simulink model "Main1"  (R2017b)
settings: Solver=ode15s  StartTime=0.0  StopTime=t_end  FixedStep=.0001  MaxStep=st  RelTol=1e-3  EnableMultiTasking=on
values from neighbouring files (symbols this model uses):
  A = eye(16,16)    [full_input_list.m]
  B = zeros(16,1)    [full_input_list.m]
  C = blkdiag(eye(3,3),zeros(3,3),eye(10,10))    [full_input_list.m]
  deltaT = 0.00001    (= 1e-05)    [full_input_list.m]
  H = C    [full_input_list.m]
  I_UD = [0.032808359, 0.000617048, 0.000049185;      0.000617048, 0.032531573, 0.000060042;      0.000049185, 0.000060042, 0.007799591]    [full_input_list.m]
  kd = 0.5    [full_input_list.m]    (also in initACS.m = 0.01)
  kd_UD_detumble = 6e-3    (= 0.006)    [full_input_list.m]
  kd_UD_slew = epsilon_UD_slew*.3    (= 0.003)    [full_input_list.m]
  kd_UD_spinUp = epsilon_UD_spinUp*0.025    (= 0.00025)    [full_input_list.m]
  kp = 1    [full_input_list.m]    (also in initACS.m = 0.01)
  kp_UD_slew = epsilon_UD_slew^2*.01    (= 1e-06)    [full_input_list.m]
  kp_UD_spinUp = epsilon_UD_spinUp^2*.05    (= 5e-06)    [full_input_list.m]
  magMomentMax_B = sat2CoilArea.*sat2n.*currentMax_B    [full_input_list.m]
  omega_cmd_N = 1e-1*[1 1 -.6]'    [full_input_list.m]
  omega_spinUp_MAG = 0.05    [full_input_list.m]
  OpModes = [0 0 0]    [full_input_list.m]
  OpTimes = [0 1 2]    [full_input_list.m]
  q4_cmd_init = [q4_cmd_init(2:4); q4_cmd_init(1)]    [full_input_list.m]
  Q_k = zeros(16,16)    [full_input_list.m]
  R = R_k    [full_input_list.m]
  sat2CoilArea = 0.8*[0.02; 0.02; 0.01]    [full_input_list.m]
  sat2n = [0; 100; 100]    [full_input_list.m]
  sat2Resistance = sat2WireLength.*sat2WireResistivity./sat2WireArea    [full_input_list.m]
  SeperationTime = 30000    [full_input_list.m]
  spinAxis_B = [1 0 0]    [full_input_list.m]
  st = 1/freq    (= 0.0125)    [full_input_list.m]    (also in initSimulink.m)
  u_k = zeros(16,1)    [full_input_list.m]
  w_k = zeros(16,1)    [full_input_list.m]
  Z_k = zeros(16,1)    [full_input_list.m]
undefined symbols (not defined in the file or in its folder): DiscIntNeverNeededParam, G_igrf, gyro_DCM_BS, H_igrf, I_B, IAU, Kschmidt, mag_variance, R_mean
libraries: aerolibutil x36, vrlib x31, SimMainLibrary x27, simulink x22, dspmathops x6, sharedtransform x4, sharedutil x2, dspinverses x2, dspmtrx3 x1, aerolibtransform2 x1, aerolibgravity2 x1, lib_violet_env x1
(part 3 of 3)

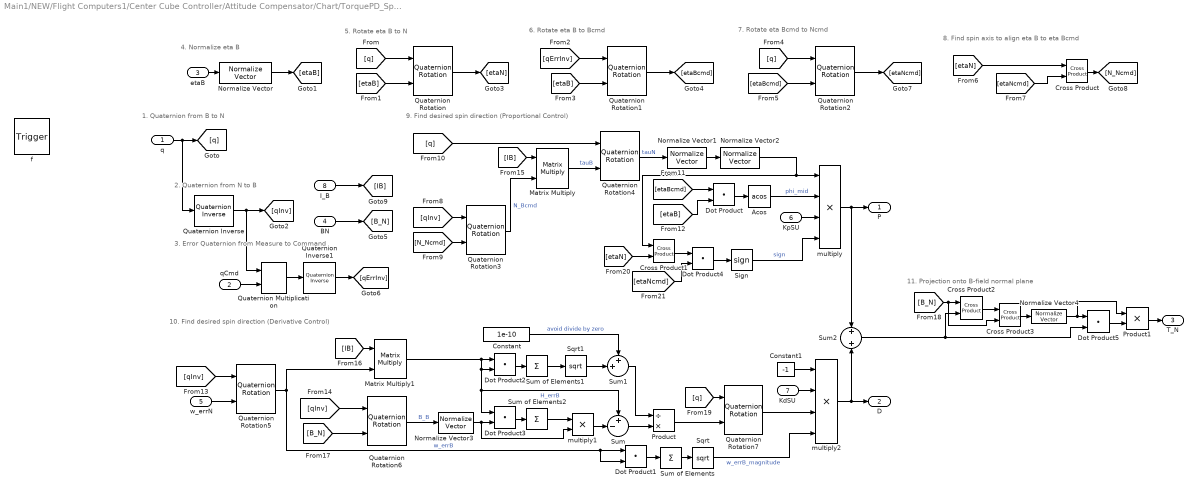
== system Main1/NEW/Flight Computers1/Center Cube Controller/Attitude Compensator/Chart/TorquePD_SpinUp ==
  note: 1. Quaternion from B to N
  note: 5. Rotate eta B to N
  note: 2. Quaternion from N to B
  note: 3. Error Quaternion from Measure to Command
  note: 6. Rotate eta B to Bcmd
  note: 7. Rotate eta Bcmd to Ncmd
  note: 8. Find spin axis to align eta B to eta Bcmd
  note: 9. Find desired spin direction (Proportional Control)
  note: 10. Find desired spin direction (Derivative Control)
  note: 4. Normalize eta B
  note: 11. Projection onto B-field normal plane
  q : Inport
  qCmd : Inport  Port=2
  etaB : Inport  Port=3
  BN : Inport  Port=4
  w_errN : Inport  Port=5
  KpSU : Inport  Port=6
  KdSU : Inport  Port=7
  I_B : Inport  Port=8
  f : TriggerPort  TriggerType=function-call  VariantControl=(inherit)
      settings: CopyFcn=Stateflow.SLINSF.SimulinkMan.removeBlockPreDeleteFcn  PreDeleteFcn=Stateflow.SLINSF.SimulinkMan.unsafePredeleteFcn
  Acos : Trigonometry  Operator=acos
  Constant : Constant  Value=1e-10
  Constant1 : Constant  Value=-1
  Cross Product{,1..3} (4 alike) : vrlib/Utilities/Cross Product
      settings: SourceProductBaseCode=VR
  Dot Product{,1..5} (6 alike) : DotProduct  InputSameDT=on  OutDataTypeStr=Inherit: Inherit via internal rule
  Matrix Multiply : Product  Multiplication=Matrix(*)
  Matrix Multiply1 : Product  Multiplication=Matrix(*)
  Normalize Vector{,1..4} (5 alike) : vrlib/Utilities/Normalize Vector  maxzero=0
      settings: SourceProductName=Simulink 3D Animation  SourceProductBaseCode=VR
  Product : Product  Inputs=/*
  Product1 : Product
  Quaternion Inverse : aerolibutil/Quaternion Inverse
      settings: SourceProductName=Aerospace Blockset
  Quaternion Inverse1 : aerolibutil/Quaternion Inverse
      settings: SourceProductName=Aerospace Blockset
  Quaternion Multiplication : aerolibutil/Quaternion Multiplication
  Quaternion Rotation{,1..7} (8 alike) : aerolibutil/Quaternion Rotation
  Sign : Signum
  Sqrt : Sqrt  SaturateOnIntegerOverflow=on
  Sqrt1 : Sqrt  SaturateOnIntegerOverflow=on
  Sum : Sum  Inputs=+-|
  Sum of Elements : Sum  Inputs=+
  Sum of Elements1 : Sum  Inputs=+
  Sum of Elements2 : Sum  Inputs=+
  Sum1 : Sum  Inputs=++|
  Sum2 : Sum
  multiply : Product  Inputs=****
  multiply1 : Product  Inputs=**
  multiply2 : Product  Inputs=****
  P : Outport
  D : Outport  Port=2
  T_N : Outport  Port=3
  wires:
  etaB/1 -> Normalize Vector/1
  Quaternion Rotation/1 -> [etaN]
  q/1 -> [q], Quaternion Inverse/1
  [q] -> Quaternion Rotation/1
  Normalize Vector/1 -> [etaB]
  [etaB] -> Quaternion Rotation/2
  Quaternion Inverse/1 -> Quaternion Multiplication/1, [qInv]
  [qErrInv] -> Quaternion Rotation1/1
  [etaB] -> Quaternion Rotation1/2
  Quaternion Rotation1/1 -> [etaBcmd]
  qCmd/1 -> Quaternion Multiplication/2
  Quaternion Multiplication/1 -> Quaternion Inverse1/1
  Quaternion Inverse1/1 -> [qErrInv]
  [q] -> Quaternion Rotation2/1
  [etaBcmd] -> Quaternion Rotation2/2
  Quaternion Rotation2/1 -> [etaNcmd]
  [etaN] -> Cross Product/1
  [etaNcmd] -> Cross Product/2
  Cross Product/1 -> [N_Ncmd]
  Quaternion Rotation3/1 -> Matrix Multiply/2  "N_Bcmd"
  [N_Ncmd] -> Quaternion Rotation3/2
  [qInv] -> Quaternion Rotation3/1
  [q] -> Quaternion Rotation4/1
  Matrix Multiply/1 -> Quaternion Rotation4/2  "tauB"
  Quaternion Rotation4/1 -> Normalize Vector1/1  "tauN"
  Normalize Vector1/1 -> Normalize Vector2/1
  Normalize Vector2/1 -> Cross Product1/1, multiply/1
  Dot Product/1 -> Acos/1
  [etaB] -> Dot Product/2
  [etaBcmd] -> Dot Product/1
  Acos/1 -> multiply/2  "phi_mid"
  KpSU/1 -> multiply/3
  multiply/1 -> P/1, Sum2/1
  [qInv] -> Quaternion Rotation5/1
  w_errN/1 -> Quaternion Rotation5/2
  [qInv] -> Quaternion Rotation6/1
  Quaternion Rotation6/1 -> Normalize Vector3/1  "B_B"
  I_B/1 -> [IB]
  [IB] -> Matrix Multiply/1
  [IB] -> Matrix Multiply1/1
  Quaternion Rotation5/1 -> Dot Product1/1, Dot Product1/2, Matrix Multiply1/2  "w_errB"
  Normalize Vector3/1 -> Dot Product3/2, multiply1/2
  Constant/1 -> Sum1/1  "avoid divide by zero"
  [q] -> Quaternion Rotation7/1
  Sum/1 -> Product/2
  Sum1/1 -> Product/1
  Product/1 -> Quaternion Rotation7/2
  Sqrt1/1 -> Sum1/2
  Matrix Multiply1/1 -> Sum/1, Dot Product3/1, Dot Product2/2, Dot Product2/1  "H_errB"
  Dot Product1/1 -> Sum of Elements/1
  Sum of Elements/1 -> Sqrt/1
  Sum of Elements1/1 -> Sqrt1/1
  Dot Product2/1 -> Sum of Elements1/1
  [etaN] -> Cross Product1/2
  Cross Product1/1 -> Dot Product4/1
  [etaNcmd] -> Dot Product4/2
  Dot Product4/1 -> Sign/1
  Sign/1 -> multiply/4  "sign"
  multiply1/1 -> Sum/2
  Dot Product3/1 -> Sum of Elements2/1
  Sum of Elements2/1 -> multiply1/1
  Quaternion Rotation7/1 -> multiply2/3
  KdSU/1 -> multiply2/2
  Constant1/1 -> multiply2/1
  multiply2/1 -> D/1, Sum2/2
  Sqrt/1 -> multiply2/4  "w_errB_magnitude"
  Normalize Vector4/1 -> Product1/1, Dot Product5/1
  Cross Product2/1 -> Cross Product3/1
  [B_N] -> Cross Product2/1, Cross Product3/2
  Cross Product3/1 -> Normalize Vector4/1
  Sum2/1 -> Cross Product2/2, Dot Product5/2
  Product1/1 -> T_N/1
  Dot Product5/1 -> Product1/2
  BN/1 -> [B_N]
  [B_N] -> Quaternion Rotation6/2

== system Main1/NEW/Flight Computers1/Center Cube Controller/Attitude Compensator/Commanded state/Quaternion Integration ==
  w_N : Inport
  Integrator1 : Integrator  InitialCondition=q4_cmd_init
  q_normalize : Subsystem
  qderiv : Subsystem
  q4 : Outport
  wires:
  w_N/1 -> qderiv/1(w)
  q_normalize/1(q_out) -> qderiv/2(q), q4/1
  Integrator1/1 -> q_normalize/1(q_in)
  qderiv/1(qd) -> Integrator1/1

== system Main1/NEW/Flight Computers1/Center Cube Controller/Attitude Compensator/Deployed Modes (switch)1/Default ==
  Action Port : ActionPort  ActionType=default
  Constant : Constant  Value=[ 0 0 0 ]
  Out1 : Outport
  wires:
  Constant/1 -> Out1/1

== system Main1/NEW/Flight Computers1/Center Cube Controller/Attitude Compensator/Deployed Modes (switch)1/Seek EKF Convergence ==
  Action Port : ActionPort  ActionType=case
  Constant : Constant  Value=[ 0 0 0 ]
  Out1 : Outport
  wires:
  Constant/1 -> Out1/1

== system Main1/NEW/Flight Computers1/Center Cube Controller/Attitude Compensator/Deployed Modes (switch)1/Spin-Up Slew ==
  note: Regulator
      | - q_target = [0 0 0 1]
      | - w_target = [0 0 0]
  q : Inport
  w : Inport  Port=2
  Action Port : ActionPort  ActionType=case
  Add : Sum
  Gain : Gain  Gain=-1
  Gain1 : Gain  Gain=kp
  Gain2 : Gain  Gain=-1
  Gain3 : Gain  Gain=kd
  Quaternion Inverse : aerolibutil/Quaternion Inverse
      settings: SourceProductName=Aerospace Blockset
  Quaternion Multiplication : aerolibutil/Quaternion Multiplication
  Selector : Selector  InputPortWidth=4  IndexOptions=Index vector (dialog)  Indices=[1 2 3]  OutputSizes=1
  Target q : Constant  Value=[ 0 0 0 1 ]
  tau : Outport
  wires:
  Gain2/1 -> Add/2
  Gain/1 -> Add/1
  Add/1 -> tau/1
  w/1 -> Gain3/1
  Gain3/1 -> Gain2/1
  Gain1/1 -> Gain/1
  Selector/1 -> Gain1/1
  Quaternion Multiplication/1 -> Selector/1
  Target q/1 -> Quaternion Inverse/1
  Quaternion Inverse/1 -> Quaternion Multiplication/2
  q/1 -> Quaternion Multiplication/1

== system Main1/NEW/Flight Computers1/Center Cube Controller/Attitude Compensator/Not Deployed Modes (switch)/Detumbling Slew ==
  note: Regulator
      | - q_target = [0 0 0 1]
      | - w_target = [0 0 0]
  note: Markley Regulator
      | This regulator takes the current directional quaterion vector, the target quaterion, the intertial matrix, and the current angular velocity to determine the required torque necessary to the slew.
      |
      | The equation is 7.8 listed on page 290 of Fundamentals of Spacecraft Attitude Determination and Control. The input I is currently not defined. Also important to the equation is equation 7.2
  q_BN : Inport
  w_BN : Inport  Port=2
  "Inertia " : Inport  Port=3
  Action Port : ActionPort
  3x3 Cross Product : sharedutil/3x3 Cross Product
      settings: SourceProductBaseCode=AE
  Add : Sum  Inputs=+++
  Gain : Gain  Gain=-1
  Gain1 : Gain  Gain=kp
  Gain2 : Gain  Gain=-1
  Gain3 : Gain  Gain=kd
  Gain4 : Gain  Gain=-1
  Product : Product  Multiplication=Matrix(*)
  Quaternion Inverse : aerolibutil/Quaternion Inverse
      settings: SourceProductName=Aerospace Blockset
  Quaternion Multiplication : aerolibutil/Quaternion Multiplication
  Selector : Selector  InputPortWidth=4  IndexOptions=Index vector (dialog)  Indices=[1 2 3]  OutputSizes=1
  Target q : Constant  Value=[ 0 0 0 1 ]
  tau : Outport
  wires:
  q_BN/1 -> Quaternion Multiplication/1
  Quaternion Inverse/1 -> Quaternion Multiplication/2
  Target q/1 -> Quaternion Inverse/1
  Quaternion Multiplication/1 -> Selector/1
  Selector/1 -> Gain1/1
  Gain1/1 -> Gain/1
  Gain3/1 -> Gain2/1
  w_BN/1 -> 3x3 Cross Product/1, Gain3/1, Product/2
  Add/1 -> tau/1
  Gain/1 -> Add/1
  Gain2/1 -> Add/2
  "Inertia "/1 -> Product/1
  Product/1 -> 3x3 Cross Product/2
  3x3 Cross Product/1 -> Gain4/1
  Gain4/1 -> Add/3

== system Main1/NEW/Flight Computers1/Center Cube Controller/Attitude Compensator/Not Deployed Modes (switch)/Inital Spin Up ==
  note: Regulator
      | - q_target = [0 0 0 1]
      | - w_target = [0 0 0]
  note: Markley Regulator
      | This regulator takes the current directional quaterion vector, the target quaterion, the intertial matrix, and the current angular velocity to determine the required torque necessary to the slew.
      |
      | The equation is 7.8 listed on page 290 of Fundamentals of Spacecraft Attitude Determination and Control. The input I is currently not defined. Also important to the equation is equation 7.2
  q_BN : Inport
  w : Inport  Port=2
  "I " : Inport  Port=3
  Action Port : ActionPort
  3x3 Cross Product : sharedutil/3x3 Cross Product
      settings: SourceProductBaseCode=AE
  Add : Sum  Inputs=+++
  Gain : Gain  Gain=-1
  Gain1 : Gain  Gain=kp
  Gain2 : Gain  Gain=-1
  Gain3 : Gain  Gain=kd
  Gain4 : Gain  Gain=-1
  Product : Product  Multiplication=Matrix(*)
  Quaternion Inverse : aerolibutil/Quaternion Inverse
      settings: SourceProductName=Aerospace Blockset
  Quaternion Multiplication : aerolibutil/Quaternion Multiplication
  Selector : Selector  InputPortWidth=4  IndexOptions=Index vector (dialog)  Indices=[1 2 3]  OutputSizes=1
  Target q : Constant  Value=[ 0 0 0 1 ]
  tau : Outport
  wires:
  q_BN/1 -> Quaternion Multiplication/1
  Quaternion Inverse/1 -> Quaternion Multiplication/2
  Target q/1 -> Quaternion Inverse/1
  Quaternion Multiplication/1 -> Selector/1
  Selector/1 -> Gain1/1
  Gain1/1 -> Gain/1
  Gain3/1 -> Gain2/1
  w/1 -> Product/2, 3x3 Cross Product/1, Gain3/1
  Add/1 -> tau/1
  Gain/1 -> Add/1
  Gain2/1 -> Add/2
  "I "/1 -> Product/1
  Product/1 -> 3x3 Cross Product/2
  3x3 Cross Product/1 -> Gain4/1
  Gain4/1 -> Add/3

== system Main1/NEW/Flight Computers1/Center Cube Controller/Attitude Compensator/Not Deployed Modes (switch)/Null Case1 ==
  Action Port : ActionPort
  Constant : Constant  Value=[ 0 0 0 ]
  Out1 : Outport
  wires:
  Constant/1 -> Out1/1

== system Main1/NEW/Flight Computers1/Center Cube Controller/Attitude Compensator/Not Deployed Modes (switch)/Seek EKF Convergence ==
  Action Port : ActionPort
  Constant : Constant  Value=[ 0 0 0 ]
  Out1 : Outport
  wires:
  Constant/1 -> Out1/1

== system Main1/NEW/Flight Computers1/Center Cube Controller/Attitude Compensator/Not Deployed Modes (switch)/Sun Pointing ==
  note: Regulator
      | - q_target = [0 0 1 0]
      | - w_target = [0 0 0]
  q : Inport
  w_BN : Inport  Port=2
  Action Port : ActionPort
  Add : Sum
  Add1 : Sum  Inputs=+-
  Gain : Gain  Gain=-1
  Gain1 : Gain  Gain=kp
  Gain2 : Gain  Gain=-1
  Gain3 : Gain  Gain=kd
  Quaternion Inverse : aerolibutil/Quaternion Inverse
      settings: SourceProductName=Aerospace Blockset
  Quaternion Multiplication : aerolibutil/Quaternion Multiplication
  Selector : Selector  InputPortWidth=4  IndexOptions=Index vector (dialog)  Indices=[1 2 3]  OutputSizes=1
  Target q : Constant  Value=[ 0 0 1 0 ]
  Target w : Constant  Value=[ 0 0 0 ]
  tau : Outport
  wires:
  q/1 -> Quaternion Multiplication/1
  Quaternion Inverse/1 -> Quaternion Multiplication/2
  Target q/1 -> Quaternion Inverse/1
  Quaternion Multiplication/1 -> Selector/1
  Selector/1 -> Gain1/1
  Gain1/1 -> Gain/1
  Gain3/1 -> Gain2/1
  w_BN/1 -> Add1/1
  Add/1 -> tau/1
  Gain/1 -> Add/1
  Gain2/1 -> Add/2
  Target w/1 -> Add1/2
  Add1/1 -> Gain3/1

== system Main1/NEW/Flight Computers1/Center Cube Controller/Attitude Compensator/Undeployed Control Modes/Change of Basis Matrix ==
  I_B : Inport
  quat1 : Inport  Port=2
  Display : Display
  Display3 : Display
  Math Function : Math  Operator=transpose  SaturateOnIntegerOverflow=on
  Product : Product  Multiplication=Matrix(*)
  Product1 : Product  Multiplication=Matrix(*)
  Q_B_N : Display
  Quaternions to Direction Cosine Matrix : sharedtransform/Quaternions to  Direction Cosine Matrix
      settings: SourceProductName=Aerospace Blockset  SourceProductBaseCode=AE
  Scope : Scope
  I_N : Outport
  wires:
  quat1/1 -> Quaternions to Direction Cosine Matrix/1, Scope/1
  Product1/1 -> Display/1, I_N/1
  I_B/1 -> Product/1, Display3/1
  Quaternions to Direction Cosine Matrix/1 -> Product/2, Math Function/1, Q_B_N/1
  Product/1 -> Product1/2
  Math Function/1 -> Product1/1

== system Main1/NEW/Flight Computers1/Center Cube Controller/Attitude Compensator/Undeployed Control Modes/Detumbling ==
  note: Regulator
      | - q_target = <input>
      | - w_target = [0 0 0]
  note: Markley Regulator
      | This regulator takes the current directional quaterion vector, the target quaterion, the intertial matrix, and the current angular velocity to determine the required torque necessary to the slew.
      |
      | The equation is 7.8 listed on page 290 of Fundamentals of Spacecraft Attitude Determination and Control. The input I is currently not defined. Also important to the equation is equation 7.2
  note: Derivative Controller
      | This controller is a pure derivative controller. It calculates torque to purely oppose the angular velocity. It is better behaved in the short-run than a PD controller projected onto the B field normal plane, but it does not allow for a quaternion command, only a detumble to an unknown attitude.
  w_BN_N : Inport
  I_N : Inport  Port=2
  Action Port : ActionPort  ActionType=case
  Gain3 : Gain  Gain=kd_UD_detumble
  Gain5 : Gain  Gain=-1
  Gain6 : Gain  Commented=on  Gain=1/I_B(1,1)
  Product2 : Product  Multiplication=Matrix(*)
  torque_N : Outport
  wires:
  Product2/1 -> Gain5/1
  Gain3/1 -> torque_N/1  "torque_N"
  I_N/1 -> Product2/1  "I_N"
  w_BN_N/1 -> Product2/2  "w_BN_N"
  Gain5/1 -> Gain3/1

== system Main1/NEW/Flight Computers1/Center Cube Controller/Attitude Compensator/Undeployed Control Modes/Null Case1 ==
  Action Port : ActionPort  ActionType=default
  Constant : Constant  Value=[ 0 0 0 ]
  Out1 : Outport
  wires:
  Constant/1 -> Out1/1

== system Main1/NEW/Flight Computers1/Center Cube Controller/Attitude Compensator/Undeployed Control Modes/Projection to B-field normal plane ==
  torque_raw_N : Inport
  B_N : Inport  Port=2
  Cross Product : vrlib/Utilities/Cross Product
      settings: SourceProductBaseCode=VR
  Cross Product1 : vrlib/Utilities/Cross Product
      settings: SourceProductBaseCode=VR
  Dot Product : DotProduct  InputSameDT=on  OutDataTypeStr=Inherit: Inherit via internal rule
  Normalize Vector : vrlib/Utilities/Normalize Vector  maxzero=0
      settings: SourceProductName=Simulink 3D Animation  SourceProductBaseCode=VR
  Product : Product
  torque_proj_N : Outport
  wires:
  Cross Product1/1 -> Normalize Vector/1
  B_N/1 -> Cross Product1/2, Cross Product/1
  Cross Product/1 -> Cross Product1/1
  Dot Product/1 -> Product/2
  torque_raw_N/1 -> Dot Product/2, Cross Product/2
  Product/1 -> torque_proj_N/1
  Normalize Vector/1 -> Product/1, Dot Product/1

== system Main1/NEW/Flight Computers1/Center Cube Controller/Attitude Compensator/Undeployed Control Modes/Quat Error1 ==
  q4_command : Inport
  q4 : Inport  Port=2
  Quat Inverse : Subsystem
  Quat product : Subsystem
  q4_error : Outport
  wires:
  Quat product/1(q_a*q_b) -> q4_error/1
  Quat Inverse/1(q_inv) -> Quat product/2(q_b)
  q4/1 -> Quat product/1(q_a)
  q4_command/1 -> Quat Inverse/1(q)

== system Main1/NEW/Flight Computers1/Center Cube Controller/Attitude Compensator/Undeployed Control Modes/Seek EKF Convergence ==
  Action Port : ActionPort  ActionType=case
  Constant : Constant  Value=[ 0 0 0 ]
  Out1 : Outport
  wires:
  Constant/1 -> Out1/1

== system Main1/NEW/Flight Computers1/Center Cube Controller/Attitude Compensator/Undeployed Control Modes/Slewing1 ==
  note: These blocks are to tell Simulink what dimensions your signal is. They help when it throws errors for mismatched dimensions when you know the dimensions are correct.
  note: Slew Maneuver Controller
      | This slew maneuver controller is used when moving from a state with small omega to an aligned axis state, spinning slowly with the spacecraft commanded spin axis in the desired inertial direction.
  q1 : Inport
  w_BN_N : Inport  Port=2
  q1_cmd : Inport  Port=3
  omegaCmd_N : Inport  Port=4
  I_B : Inport  Port=5
  B_N : Inport  Port=6
  Action Port : ActionPort  ActionType=case
  Constant : Constant  Value=kp_UD_slew
  Constant1 : Constant  Value=kd_UD_slew
  Control Components : Scope  NumInputPorts=2
  Gain : Gain  Gain=omega_spinUp_MAG
  Gain6 : Gain
  MATLAB Function : Subsystem  TreatAsAtomicUnit=on
  Normalize Vector : vrlib/Utilities/Normalize Vector  maxzero=0
      settings: SourceProductName=Simulink 3D Animation  SourceProductBaseCode=VR
  Signal Specification : SignalSpecification  OutDataTypeStr=double  Dimensions=3
  Signal Specification1 : SignalSpecification  OutDataTypeStr=double  Dimensions=3
  Sum : Sum  Inputs=|++
  Sum1 : Sum  Inputs=|+-
  eta_B1 : Constant  Value=spinAxis_B
  torque_N : Outport
  wires:
  q1/1 -> MATLAB Function/1(quat1)
  q1_cmd/1 -> MATLAB Function/2(quat1_cmd)
  I_B/1 -> MATLAB Function/8(I_B)
  eta_B1/1 -> MATLAB Function/3(eta_B)
  B_N/1 -> MATLAB Function/4(B_N)
  Sum/1 -> torque_N/1
  MATLAB Function/1(torqueP_N) -> Signal Specification1/1  "torqueP_N"
  MATLAB Function/2(torqueD_N) -> Signal Specification/1  "torqueD_N"
  Gain6/1 -> Sum/1
  Sum1/1 -> MATLAB Function/5(omegaErr_N)
  w_BN_N/1 -> Sum1/1
  Signal Specification/1 -> Control Components/2, Sum/2
  Constant/1 -> MATLAB Function/6(kp)
  Constant1/1 -> MATLAB Function/7(kd)
  Signal Specification1/1 -> Control Components/1, Gain6/1
  omegaCmd_N/1 -> Normalize Vector/1
  Normalize Vector/1 -> Gain/1
  Gain/1 -> Sum1/2

== system Main1/NEW/Flight Computers1/Center Cube Controller/Attitude Compensator/Undeployed Control Modes/Spin-up ==
  note: Regulator
      | - q_target = <input>
      | - w_target = [0 0 0]
  note: Slew Maneuver Controller
      | This slew maneuver controller is used when moving from a state with small omega to a static attitude command. This is used primarily to set up the spacecraft with the desired body spin axis aligned with the desired inertial spin axis.
  q1 : Inport
  w_BN_N : Inport  Port=2
  q1_cmd : Inport  Port=3
  omegaCmd_N : Inport  Port=4
  I_B : Inport  Port=5
  B_N : Inport  Port=6
  Action Port : ActionPort  ActionType=case
  Constant : Constant  Value=kp_UD_spinUp
  Constant1 : Constant  Value=kd_UD_spinUp
  Control Components : Scope  NumInputPorts=2
  Display : Display
  Display1 : Display
  Gain6 : Gain
  MATLAB Function : Subsystem  TreatAsAtomicUnit=on
  Signal Specification : SignalSpecification  OutDataTypeStr=double  Dimensions=3
  Signal Specification1 : SignalSpecification  OutDataTypeStr=double  Dimensions=3
  Signal Specification2 : SignalSpecification  OutDataTypeStr=double  Dimensions=1
  Signal Specification3 : SignalSpecification  OutDataTypeStr=double  Dimensions=1
  Sum : Sum  Inputs=|++
  Sum1 : Sum  Inputs=|+-
  eta_B1 : Constant  Value=spinAxis_B
  torque_N : Outport
  wires:
  q1/1 -> MATLAB Function/1(quat1)
  q1_cmd/1 -> MATLAB Function/2(quat1_cmd)
  I_B/1 -> MATLAB Function/8(I_B)
  eta_B1/1 -> MATLAB Function/3(eta_B)
  B_N/1 -> MATLAB Function/4(B_N)
  Constant/1 -> Signal Specification2/1
  Constant1/1 -> Signal Specification3/1
  Sum/1 -> torque_N/1
  MATLAB Function/1(torqueP_N) -> Signal Specification1/1  "torqueP_N"
  MATLAB Function/2(torqueD_N) -> Signal Specification/1  "torqueD_N"
  Gain6/1 -> Sum/1
  Sum1/1 -> MATLAB Function/5(omegaErr_N)
  w_BN_N/1 -> Sum1/1
  omegaCmd_N/1 -> Sum1/2
  Signal Specification/1 -> Control Components/2, Display1/1, Sum/2  "torqueD_N"
  Signal Specification1/1 -> Display/1, Control Components/1, Gain6/1  "torqueP_N"
  Signal Specification2/1 -> MATLAB Function/6(kp)
  Signal Specification3/1 -> MATLAB Function/7(kd)

== system Main1/NEW/Flight Computers1/Center Cube Controller/Torque Coil Management/Torque Coil Management/Magnetic Moment Direction ==
  note: Aperp_B is the normal vector to the plane of attainable magnetic moments by the 2 coils in the b2 and b3 directions
  torque_cmd_N : Inport
  q4 : Inport  Port=2
  Aperp_B : Constant  Value=[1;0;0]
  Change of Basis1 : SimMainLibrary/Change of Basis1
      settings: SourceProductName=CUGravity Library
  Cross Product : vrlib/Utilities/Cross Product
      settings: SourceProductBaseCode=VR
  Display : Display  Commented=on
  Normalize Vector : vrlib/Utilities/Normalize Vector  maxzero=0
      settings: SourceProductName=Simulink 3D Animation  SourceProductBaseCode=VR
  Signal Specification1 : SignalSpecification  OutDataTypeStr=double  Dimensions=3
  muHat_B : Outport
  wires:
  Change of Basis1/1 -> Display/1, Cross Product/2  "torque_B"
  torque_cmd_N/1 -> Change of Basis1/1
  Normalize Vector/1 -> Signal Specification1/1  "muHat_B"
  Aperp_B/1 -> Cross Product/1
  q4/1 -> Change of Basis1/2
  Cross Product/1 -> Normalize Vector/1
  Signal Specification1/1 -> muHat_B/1

== system Main1/NEW/Flight Computers1/Center Cube Controller/Torque Coil Management/Torque Coil Management/Magnetic moment Magnitude ==
  note: Singularity aviodance algorithm is flawed. Need to redo.
  torque_cmd_N : Inport
  muHat_B : Inport  Port=2
  B_B : Inport  Port=3
  Acos : Trigonometry  Operator=acos
  Add : Sum
  Avoid singularity : Constant  Value=0
  Display : Display
  Divide : Product  Inputs=*//
  Dot Product : DotProduct  InputSameDT=on  OutDataTypeStr=Inherit: Inherit via internal rule
  Normalize Vector1 : vrlib/Utilities/Normalize Vector  maxzero=0
      settings: SourceProductName=Simulink 3D Animation  SourceProductBaseCode=VR
  Sin : Trigonometry
  Vector Magnitude : SimMainLibrary/Vector Magnitude
      settings: SourceProductName=CUGravity Library
  Vector Magnitude1 : SimMainLibrary/Vector Magnitude
      settings: SourceProductName=CUGravity Library
  ||mu|| : Outport
  wires:
  Vector Magnitude1/1 -> Divide/3
  Dot Product/1 -> Acos/1
  Divide/1 -> ||mu||/1
  torque_cmd_N/1 -> Vector Magnitude/1
  B_B/1 -> Vector Magnitude1/1, Normalize Vector1/1
  muHat_B/1 -> Dot Product/1
  Sin/1 -> Display/1, Add/1
  Acos/1 -> Sin/1
  Vector Magnitude/1 -> Divide/1
  Avoid singularity/1 -> Add/2
  Add/1 -> Divide/2
  Normalize Vector1/1 -> Dot Product/2

== system Main1/NEW/Flight Computers1/Center Cube Controller/Torque Coil Management/Torque Coil Management/Reduce Wasted Effort ==
  note: Reduce Wasted Effort
      | Author: Aaron Sandoval
      | This function detects how close the direction of the commanded mag. moment is to the external magnetic field. If it is very close, then the resulting torque will be minimal, and a lot of energy is expelled for little torque. A nonlinear, continuous gain is applied which drives the torque to zero near alignment, and preserves the value otherwise.
  muHat_B : Inport
  mu_sat_B : Inport  Port=2
  B_B : Inport  Port=3
  Constant2 : Constant  Value=100
  Dot Product : DotProduct  InputSameDT=on  OutDataTypeStr=Inherit: Inherit via internal rule
  Fcn : Fcn  Expr=1-exp(-u(2)*(u(1)+1)^2)-exp(-u(2)*(u(1)-1)^2)
  Mux2 : Mux  Inputs=2
  Normalize Vector : vrlib/Utilities/Normalize Vector  maxzero=0
      settings: SourceProductName=Simulink 3D Animation  SourceProductBaseCode=VR
  Product1 : Product
  Ramp : simulink/Sources/Ramp  Commented=on  slope=1  start=0  X0=-2
  Scope : Scope
  mu_sat_B1 : Outport
  wires:
  mu_sat_B/1 -> Product1/1
  muHat_B/1 -> Dot Product/1
  B_B/1 -> Normalize Vector/1
  Mux2/1 -> Fcn/1
  Constant2/1 -> Mux2/2
  Fcn/1 -> Scope/1, Product1/2  "mu_sat_B"
  Product1/1 -> mu_sat_B1/1  "mu_sat_B"
  Dot Product/1 -> Mux2/1
  Normalize Vector/1 -> Dot Product/2

== system Main1/NEW/Flight Computers1/Center Cube Controller/Torque Coil Management/Torque Coil Management/Sign of torqueHat ==
  torque_cmd_N : Inport
  torque_N : Inport  Port=2
  Math Function : Math  Operator=transpose  SaturateOnIntegerOverflow=on
  Product1 : Product  Multiplication=Matrix(*)
  Sign : Signum
  Sign_B & mu : Outport
  wires:
  Math Function/1 -> Product1/1
  Sign/1 -> Sign_B & mu/1
  torque_cmd_N/1 -> Math Function/1
  torque_N/1 -> Product1/2
  Product1/1 -> Sign/1

== system Main1/NEW/Flight Computers1/Center Cube Controller/Torque Coil Management/Torque Coil Management/Subsystem ==
  mu_B23 : Inport
  Constant : Constant  Value=0
  Demux : Demux  Outputs=2
  Mux : Mux  Inputs=3
  mu_B : Outport
  wires:
  mu_B23/1 -> Demux/1
  Constant/1 -> Mux/1
  Mux/1 -> mu_B/1  "mu_B"
  Demux/1 -> Mux/2
  Demux/2 -> Mux/3

== system Main1/NEW/Flight Computers1/CenterCube EKF/New State Prediction /A_LKF/MATLAB Function ==
  "A " : Inport
  replacement : Inport  Port=2
  " Demux " : Demux  Outputs=1
  " SFunction " : S-Function  Tag=Stateflow S-Function Main 15  FunctionName=sf_sfun  PortCounts=[2 2]  SFunctionDeploymentMode=off  EnableBusSupport=on
  " Terminator " : Terminator
  A : Outport
  wires:
  "A "/1 -> " SFunction "/1
  replacement/1 -> " SFunction "/2
  " SFunction "/2 -> A/1  "A"
  " Demux "/1 -> " Terminator "/1
  " SFunction "/1 -> " Demux "/1

== system Main1/NEW/Flight Computers1/CenterCube EKF/x_measured/Lookup Tables/GPS time to Jd sfrom J2000 ==
  In1 : Inport
  Jd since GPS0 : Constant  Value=2444244.5
  Jd since J2000 : Constant  Value=2451545
  "Leap Seconds from GSP0 " : Constant  Value=27-9
  Sum : Sum  Inputs=|++
  Sum1 : Sum  Inputs=|++
  Sum2 : Sum  Inputs=|+-
  seconds to days conversion : Gain  Gain=1/86400
  Out1 : Outport
  wires:
  In1/1 -> Sum/1
  "Leap Seconds from GSP0 "/1 -> Sum/2
  Sum/1 -> seconds to days conversion/1
  seconds to days conversion/1 -> Sum1/1
  Jd since GPS0/1 -> Sum1/2
  Sum1/1 -> Sum2/1
  Jd since J2000/1 -> Sum2/2
  Sum2/1 -> Out1/1

== system Main1/NEW/Flight Computers1/CenterCube EKF/x_measured/Lookup Tables/Sun position off of Jd frm J2000 ==
  In1 : Inport
  Gain : Gain  Gain=1.49597871e8
  MATLAB Function : Subsystem  TreatAsAtomicUnit=on
  Out1 : Outport
  wires:
  In1/1 -> MATLAB Function/1(J2000_days)
  MATLAB Function/1(S_ECI) -> Gain/1
  Gain/1 -> Out1/1

== system Main1/NEW/Flight Computers1/CenterCube EKF/x_measured/q_N from Sensors/quat From DCM ==
  Q : Inport
  " Demux " : Demux  Outputs=1
  " SFunction " : S-Function  Tag=Stateflow S-Function Main 18  FunctionName=sf_sfun  PortCounts=[1 3]  SFunctionDeploymentMode=off  EnableBusSupport=on
  " Terminator " : Terminator
  q_N : Outport
  D : Outport  Port=2
  wires:
  Q/1 -> " SFunction "/1
  " SFunction "/2 -> q_N/1  "q_N"
  " SFunction "/3 -> D/1  "D"
  " Demux "/1 -> " Terminator "/1
  " SFunction "/1 -> " Demux "/1

== system Main1/NEW/Sensors1/Center Cube Sensors/Create Sun Vector/Sun position off of Jd frm J2000/MATLAB Function ==
  J2000_days : Inport
  " Demux " : Demux  Outputs=1
  " SFunction " : S-Function  Tag=Stateflow S-Function Main 21  FunctionName=sf_sfun  PortCounts=[1 2]  SFunctionDeploymentMode=off  EnableBusSupport=on
  " Terminator " : Terminator
  S_ECI : Outport
  wires:
  J2000_days/1 -> " SFunction "/1
  " SFunction "/2 -> S_ECI/1  "S_ECI"
  " Demux "/1 -> " Terminator "/1
  " SFunction "/1 -> " Demux "/1

== system Main1/NEW/Flight Computers1/Center Cube Controller/Attitude Compensator/Commanded state/Quaternion Integration/q_normalize ==
  q_in : Inport  PortDimensions=4
  Dot Product : DotProduct  InputSameDT=on  OutDataTypeStr=Inherit: Inherit via internal rule
  Math Function : Math  Operator=sqrt  SaturateOnIntegerOverflow=on
  Product : Product  Inputs=*/  SaturateOnIntegerOverflow=on  InputSameDT=on  OutDataTypeStr=Inherit: Same as first input
  q_out : Outport
  wires:
  Product/1 -> q_out/1
  Math Function/1 -> Product/2
  Dot Product/1 -> Math Function/1
  q_in/1 -> Dot Product/2, Dot Product/1, Product/1

== system Main1/NEW/Flight Computers1/Center Cube Controller/Attitude Compensator/Commanded state/Quaternion Integration/qderiv ==
  w : Inport
  q : Inport  Port=2
  Mux : Mux  Inputs=2
  Mux1 : Mux
  qd1 : Fcn  Expr=(u(7)*u(1)-u(6)*u(2)+u(5)*u(3))/2
  qd2 : Fcn  Expr=(u(6)*u(1)+u(7)*u(2)-u(4)*u(3))/2
  qd3 : Fcn  Expr=(-u(5)*u(1)+u(4)*u(2)+u(7)*u(3))/2
  qd4 : Fcn  Expr=(-u(4)*u(1)-u(5)*u(2)-u(6)*u(3))/2
  qd : Outport
  wires:
  Mux1/1 -> qd/1
  qd4/1 -> Mux1/4
  qd3/1 -> Mux1/3
  qd2/1 -> Mux1/2
  qd1/1 -> Mux1/1
  Mux/1 -> qd4/1, qd3/1, qd2/1, qd1/1
  q/1 -> Mux/2
  w/1 -> Mux/1

== system Main1/NEW/Flight Computers1/Center Cube Controller/Attitude Compensator/Undeployed Control Modes/Quat Error1/Quat Inverse ==
  q : Inport
  Demux2 : Demux
  Gain : Gain  Gain=-1
  Mux : Mux
  q_inv : Outport
  wires:
  Gain/1 -> Mux/4
  Demux2/3 -> Mux/3
  q/1 -> Demux2/1
  Demux2/2 -> Mux/2
  Demux2/1 -> Mux/1
  Demux2/4 -> Gain/1
  Mux/1 -> q_inv/1

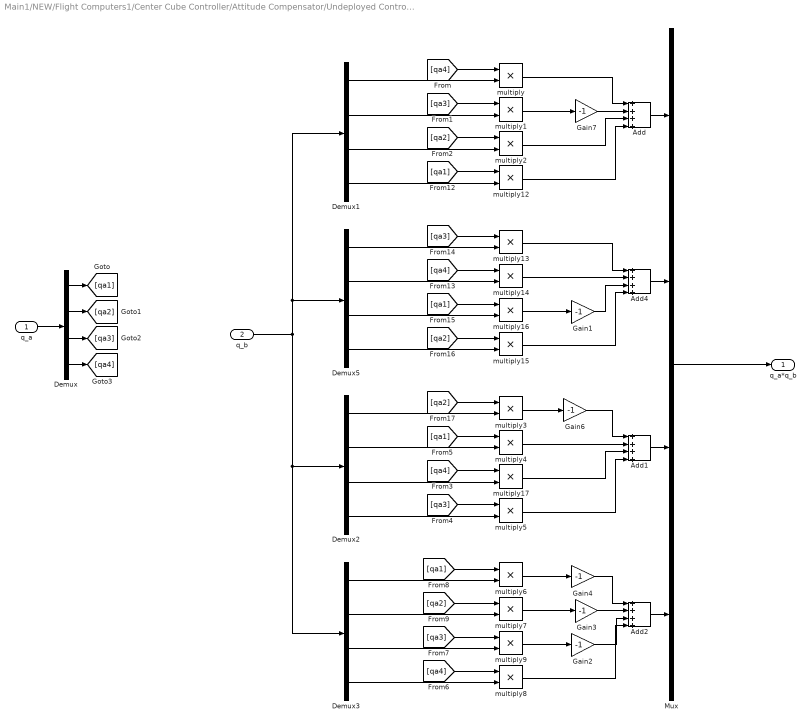
== system Main1/NEW/Flight Computers1/Center Cube Controller/Attitude Compensator/Undeployed Control Modes/Quat Error1/Quat product ==
  q_a : Inport
  q_b : Inport  Port=2
  Add{,1..2,4} (4 alike) : Sum  Inputs=++++
  Demux{,1..3,5} (5 alike) : Demux
  Gain{1..4,6..7} (6 alike) : Gain  Gain=-1
  Mux : Mux
  multiply{,1..9,12..17} (16 alike) : Product  Inputs=**
  q_a*q_b : Outport
  wires:
  q_a/1 -> Demux/1
  multiply/1 -> Add/1
  multiply2/1 -> Add/3
  Add2/1 -> Mux/4
  Add/1 -> Mux/1
  Demux1/3 -> multiply2/2
  Demux/3 -> [qa3]
  Mux/1 -> q_a*q_b/1
  Add1/1 -> Mux/3
  Demux/2 -> [qa2]
  multiply1/1 -> Gain7/1
  Demux1/2 -> multiply1/2
  Demux1/1 -> multiply/2
  Add4/1 -> Mux/2
  [qa2] -> multiply2/1
  Demux/1 -> [qa1]
  [qa3] -> multiply1/1
  Gain7/1 -> Add/2
  [qa4] -> multiply/1
  Demux/4 -> [qa4]
  [qa1] -> multiply12/1
  multiply12/1 -> Add/4
  Demux1/4 -> multiply12/2
  [qa3] -> multiply13/1
  multiply14/1 -> Add4/2
  [qa4] -> multiply14/1
  Demux5/1 -> multiply13/2
  [qa1] -> multiply16/1
  Demux5/2 -> multiply14/2
  multiply16/1 -> Gain1/1
  multiply13/1 -> Add4/1
  multiply15/1 -> Add4/4
  Demux5/4 -> multiply15/2
  Demux5/3 -> multiply16/2
  [qa2] -> multiply15/1
  Gain1/1 -> Add4/3
  [qa2] -> multiply3/1
  multiply17/1 -> Add1/3
  [qa4] -> multiply17/1
  [qa1] -> multiply4/1
  multiply5/1 -> Add1/4
  Demux2/3 -> multiply17/2
  Demux2/4 -> multiply5/2
  Demux2/2 -> multiply4/2
  Demux2/1 -> multiply3/2
  [qa3] -> multiply5/1
  multiply4/1 -> Add1/2
  multiply3/1 -> Gain6/1
  Gain6/1 -> Add1/1
  [qa1] -> multiply6/1
  q_b/1 -> Demux3/1, Demux2/1, Demux1/1, Demux5/1
  Gain2/1 -> Add2/3
  [qa3] -> multiply9/1
  [qa2] -> multiply7/1
  multiply8/1 -> Add2/4
  Demux3/3 -> multiply9/2
  Demux3/4 -> multiply8/2
  Demux3/2 -> multiply7/2
  Demux3/1 -> multiply6/2
  [qa4] -> multiply8/1
  multiply7/1 -> Gain3/1
  multiply9/1 -> Gain2/1
  multiply6/1 -> Gain4/1
  Gain4/1 -> Add2/1
  Gain3/1 -> Add2/2

== system Main1/NEW/Flight Computers1/Center Cube Controller/Attitude Compensator/Undeployed Control Modes/Slewing1/MATLAB Function ==
  quat1 : Inport
  quat1_cmd : Inport  Port=2
  eta_B : Inport  Port=3
  B_N : Inport  Port=4
  omegaErr_N : Inport  Port=5
  kp : Inport  Port=6
  kd : Inport  Port=7
  I_B : Inport  Port=8
  " Demux " : Demux  Outputs=1
  " SFunction " : S-Function  Tag=Stateflow S-Function Main 6  FunctionName=sf_sfun  PortCounts=[8 3]  SFunctionDeploymentMode=off  EnableBusSupport=on
  " Terminator " : Terminator
  torqueP_N : Outport
  torqueD_N : Outport  Port=2
  wires:
  quat1/1 -> " SFunction "/1
  quat1_cmd/1 -> " SFunction "/2
  eta_B/1 -> " SFunction "/3
  B_N/1 -> " SFunction "/4
  omegaErr_N/1 -> " SFunction "/5
  kp/1 -> " SFunction "/6
  kd/1 -> " SFunction "/7
  I_B/1 -> " SFunction "/8
  " SFunction "/2 -> torqueP_N/1  "torqueP_N"
  " SFunction "/3 -> torqueD_N/1  "torqueD_N"
  " Demux "/1 -> " Terminator "/1
  " SFunction "/1 -> " Demux "/1

== system Main1/NEW/Flight Computers1/Center Cube Controller/Attitude Compensator/Undeployed Control Modes/Spin-up/MATLAB Function ==
  quat1 : Inport
  quat1_cmd : Inport  Port=2
  eta_B : Inport  Port=3
  B_N : Inport  Port=4
  omegaErr_N : Inport  Port=5
  kp : Inport  Port=6
  kd : Inport  Port=7
  I_B : Inport  Port=8
  " Demux " : Demux  Outputs=1
  " SFunction " : S-Function  Tag=Stateflow S-Function Main 11  FunctionName=sf_sfun  PortCounts=[8 3]  SFunctionDeploymentMode=off  EnableBusSupport=on
  " Terminator " : Terminator
  torqueP_N : Outport
  torqueD_N : Outport  Port=2
  wires:
  quat1/1 -> " SFunction "/1
  quat1_cmd/1 -> " SFunction "/2
  eta_B/1 -> " SFunction "/3
  B_N/1 -> " SFunction "/4
  omegaErr_N/1 -> " SFunction "/5
  kp/1 -> " SFunction "/6
  kd/1 -> " SFunction "/7
  I_B/1 -> " SFunction "/8
  " SFunction "/2 -> torqueP_N/1  "torqueP_N"
  " SFunction "/3 -> torqueD_N/1  "torqueD_N"
  " Demux "/1 -> " Terminator "/1
  " SFunction "/1 -> " Demux "/1

== system Main1/NEW/Flight Computers1/CenterCube EKF/x_measured/Lookup Tables/Sun position off of Jd frm J2000/MATLAB Function ==
  J2000_days : Inport
  " Demux " : Demux  Outputs=1
  " SFunction " : S-Function  Tag=Stateflow S-Function Main 17  FunctionName=sf_sfun  PortCounts=[1 2]  SFunctionDeploymentMode=off  EnableBusSupport=on
  " Terminator " : Terminator
  S_ECI : Outport
  wires:
  J2000_days/1 -> " SFunction "/1
  " SFunction "/2 -> S_ECI/1  "S_ECI"
  " Demux "/1 -> " Terminator "/1
  " SFunction "/1 -> " Demux "/1
